simulink model "phase2_3D_path_following"  (R2017b)
settings: Solver=VariableStepAuto  StartTime=0.0  StopTime=5  RelTol=1e-3
values from neighbouring files (symbols this model uses):
  c = 1.140*10^-7    (= 1.14e-07)    [run_this_and_plot.m]
  g = 9.81    [run_this_and_plot.m]
  Ix = 4.856*10^(-3)    (= 0.004856)    [run_this_and_plot.m]
  Iy = 4.856*10^(-3)    (= 0.004856)    [run_this_and_plot.m]
  Iz = 8.801*10^(-3)    (= 0.008801)    [run_this_and_plot.m]
  k = 2.980*10^-6    (= 2.98e-06)    [run_this_and_plot.m]
  l = 0.225    [run_this_and_plot.m]
  m = 3    [run_this_and_plot.m]
libraries: simulink x3
settings Model: Creator=Administrator  LastModifiedBy=chenjiasheng
settings CodeAppCC: StateflowObjectComments=on

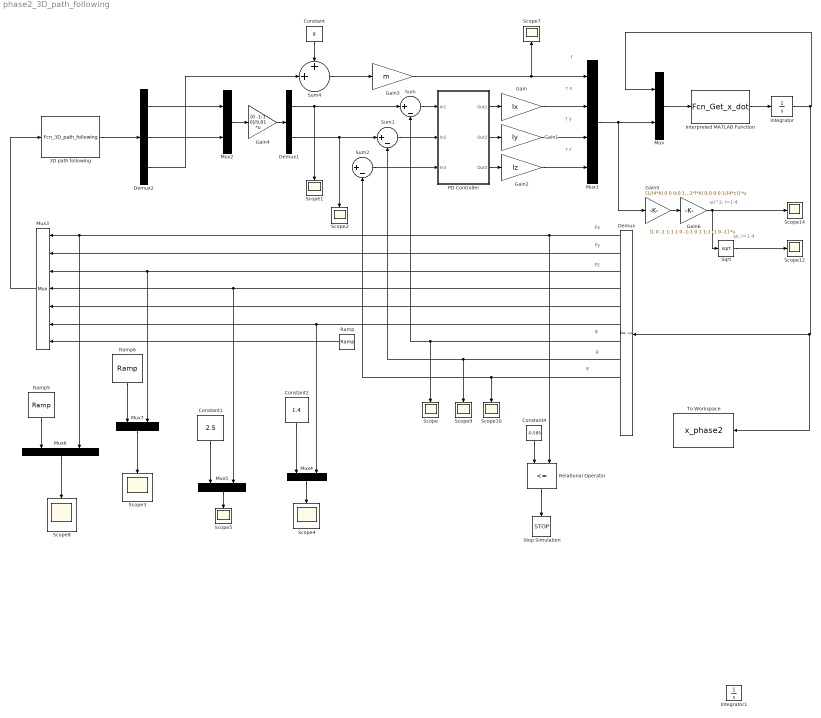
== system phase2_3D_path_following ==
  note: f
  note: τ x
  note: τ y
  note: τ z
  note: Px
  note: Py
  note: Pz
  note: φ
  note: θ
  note: ψ
  note: ωi^2, i=1-4
  note: ωi, i=1-4
  3D path following : MATLABFcn  MATLABFcn=Fcn_3D_path_following  OutputDimensions=3
  Constant : Constant  Value=g
  Constant1 : Constant  Value=2.5
  Constant2 : Constant  Value=1.4
  Constant4 : Constant  Value=-0.585
  Demux : Demux  Outputs=12
  Demux1 : Demux  Outputs=2
  Demux2 : Demux  Outputs=3
  Gain : Gain  Gain=Ix
  Gain1 : Gain  Gain=Iy
  Gain2 : Gain  Gain=Iz
  Gain3 : Gain  Gain=m
  Gain4 : Gain  Gain=[0 -1;1 0]/9.81  Multiplication=Matrix(K*u) (u vector)
  Gain5 : Gain  Gain=[1/(4*k) 0 0 0;0 1/(2*l*k) 0 0;0 0 1/(2*l*k) 0;0 0 0 1/(4*c)]  Multiplication=Matrix(K*u) (u vector)
  Gain6 : Gain  Gain=[1 0 -1 1;1 1 0 -1;1 0 1 1;1 -1 0 -1]  Multiplication=Matrix(K*u) (u vector)
  Integrator : Integrator  InitialCondition=[-4.835 0 -2.607, 0 0 0, 0 0 0, 0 0 0]
  Integrator1 : Integrator
  Interpreted MATLAB Function : MATLABFcn  MATLABFcn=Fcn_Get_x_dot  OutputDimensions=12
  Mux{,2,4..7} (6 alike) : Mux  Inputs=2
  Mux1 : Mux
  Mux3 : Mux  Inputs=7
  PD Controller : Subsystem
  Ramp : simulink/Sources/Ramp  slope=1  start=0  X0=0
  Ramp5 : simulink/Sources/Ramp  slope=2.5  start=0  X0=-4.835
  Ramp6 : simulink/Sources/Ramp  slope=1.4  start=0  X0=-2.607
  Relational Operator : RelationalOperator  Operator=<=  OutDataTypeStr=boolean  RndMeth=Nearest
  Scope{,1..5,7..10,12,14} (12 alike) : Scope
  Sqrt : Sqrt  SaturateOnIntegerOverflow=on
  Stop Simulation : Stop
  Sum : Sum  Inputs=|+-
  Sum1 : Sum  Inputs=|+-
  Sum2 : Sum  Inputs=|+-
  Sum4 : Sum  Inputs=++|
  To Workspace : ToWorkspace  VariableName=x_phase2  SampleTime=0.01
  wires:
  Mux/1 -> Interpreted MATLAB Function/1
  Interpreted MATLAB Function/1 -> Integrator/1
  Integrator/1 -> To Workspace/1, Demux/1, Mux/1
  Mux1/1 -> Gain5/1, Mux/2
  Gain/1 -> Mux1/2
  Gain1/1 -> Mux1/3
  Gain2/1 -> Mux1/4
  Demux/7 -> Scope/1, Sum/2
  Demux/8 -> Scope9/1, Sum1/2
  Demux/9 -> Scope10/1, Sum2/2
  Gain3/1 -> Mux1/1, Scope7/1
  Sum4/1 -> Gain3/1
  Constant/1 -> Sum4/1
  Mux2/1 -> Gain4/1
  Demux1/2 -> Scope2/1, Sum1/1
  Demux1/1 -> Sum/1, Scope1/1
  Gain4/1 -> Demux1/1
  Demux/1 -> Relational Operator/2, Mux3/1, Mux6/2
  Demux/2 -> Mux3/2
  Demux/3 -> Mux7/2, Mux3/3
  Demux/4 -> Mux3/4, Mux5/2
  Demux/5 -> Mux3/5
  Demux/6 -> Mux3/6, Mux4/2
  Ramp/1 -> Mux3/7
  Mux3/1 -> 3D path following/1
  3D path following/1 -> Demux2/1
  Demux2/1 -> Mux2/1
  Demux2/2 -> Mux2/2
  Demux2/3 -> Sum4/2
  Mux4/1 -> Scope4/1
  Mux5/1 -> Scope5/1
  Mux6/1 -> Scope8/1
  Mux7/1 -> Scope3/1
  Constant1/1 -> Mux5/1
  PD Controller/1(Out1) -> Gain/1
  PD Controller/2(Out2) -> Gain1/1
  PD Controller/3(Out3) -> Gain2/1
  Sum/1 -> PD Controller/1(In1)
  Sum1/1 -> PD Controller/2(In2)
  Sum2/1 -> PD Controller/3(In3)
  Gain5/1 -> Gain6/1
  Sqrt/1 -> Scope12/1
  Gain6/1 -> Sqrt/1, Scope14/1
  Ramp5/1 -> Mux6/1
  Ramp6/1 -> Mux7/1
  Constant2/1 -> Mux4/1
  Relational Operator/1 -> Stop Simulation/1
  Constant4/1 -> Relational Operator/1

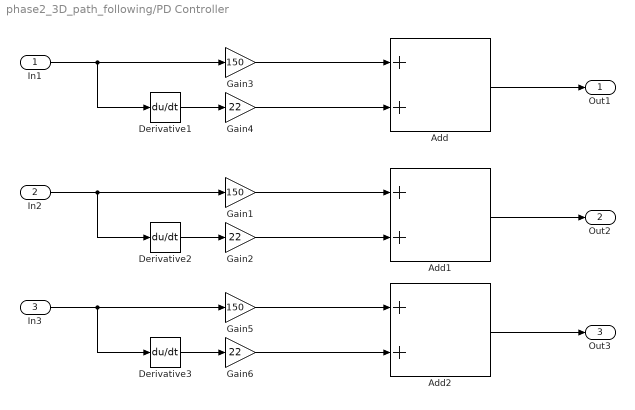
== system phase2_3D_path_following/PD Controller ==
  In1 : Inport
  In2 : Inport  Port=2
  In3 : Inport  Port=3
  Add : Sum
  Add1 : Sum
  Add2 : Sum
  Derivative1 : Derivative
  Derivative2 : Derivative
  Derivative3 : Derivative
  Gain1 : Gain  Gain=150
  Gain2 : Gain  Gain=22
  Gain3 : Gain  Gain=150
  Gain4 : Gain  Gain=22
  Gain5 : Gain  Gain=150
  Gain6 : Gain  Gain=22
  Out1 : Outport
  Out2 : Outport  Port=2
  Out3 : Outport  Port=3
  wires:
  Gain3/1 -> Add/1
  In1/1 -> Derivative1/1, Gain3/1
  Gain4/1 -> Add/2
  Derivative1/1 -> Gain4/1
  Add/1 -> Out1/1
  Add1/1 -> Out2/1
  Derivative2/1 -> Gain2/1
  Gain2/1 -> Add1/2
  In2/1 -> Gain1/1, Derivative2/1
  Gain1/1 -> Add1/1
  Gain5/1 -> Add2/1
  In3/1 -> Derivative3/1, Gain5/1
  Gain6/1 -> Add2/2
  Derivative3/1 -> Gain6/1
  Add2/1 -> Out3/1
